simulink model "REGULATORSYSTEM"  (R2019a)
settings: Solver=VariableStepAuto  StartTime=0.0  StopTime=1200  RelTol=1e-3
values from neighbouring files (symbols this model uses):
  A = [ 0 1 0 0; 0 0 1 0; 0 0 0 1;0 0 (-Ks* (M1+M2)/M1*M2) 0]    [HANDECODE.m]
  Am = Sistem.A    [HANDECODE.m]
  B = [0 0; 0 0; 0 0; 1/M1 Ks/(M1*M2)]    [HANDECODE.m]
  Bm = Sistem.B    [HANDECODE.m]
  C = [1 0 0 0]    [HANDECODE.m]
  Cm = Sistem.C    [HANDECODE.m]
  Dm = Sistem.D    [HANDECODE.m]
  K = lqr(Sistem,1,1)    [HANDECODE.m]
undefined symbols (not defined in the file or in its folder): Continuous, Time
libraries: ctrlSharedLib x1
settings Model: Creator=tr531  LastModifiedBy=tr531

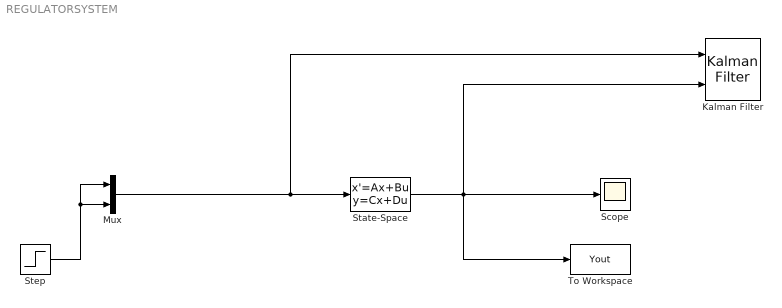
== system REGULATORSYSTEM ==
  Kalman Filter : ctrlSharedLib/Kalman Filter  TimeDomain=Continuous-Time  UseCurrentEstimator=on  ModelSource=Individual A, B, C, D matrices  ModelSourceVariable=ss(0.95,1,1,0,1)  A=A  B=B  C=C  D=[1 1]  NumberOfStates=1  NumberOfInputs=1  NumberOfOutputs=1  InitialEstimateSource=Dialog  X0=0  P0=10  UseK=off  UseGH=off  NumberOfProcessNoiseInputs=1  G=1  TimeInvariantG=on  H=0  TimeInvariantH=on  Q=1  TimeInvariantQ=on  R=1  TimeInvariantR=on  N=0  TimeInvariantN=on  AddInputPort=on  AddEnablePort=off  OutputEstimatedY=on  OutputP=off  Ts=-1
      settings: SourceProductBaseCode=CT
  Mux : Mux  Inputs=2
  Scope : Scope
  State-Space : StateSpace  A=Am-Bm*K  B=zeros(size(Bm))  C=Cm-Dm*K  D=zeros(size(Dm))  InitialCondition=[5 5 5 5]
  Step : Step  SampleTime=0
  To Workspace : ToWorkspace  VariableName=Yout  SaveFormat=Timeseries  SampleTime=-1
  wires:
  Step/1 -> Mux/2, Mux/1
  State-Space/1 -> To Workspace/1, Kalman Filter/2, Scope/1
  Mux/1 -> Kalman Filter/1, State-Space/1
